simulink model "test02"  (R2025b)
settings: Solver=VariableStepAuto  StartTime=0.0  StopTime=60  RelTol=1e-3
settings Model: Creator=sanborkl  LastModifiedBy=sanborkl

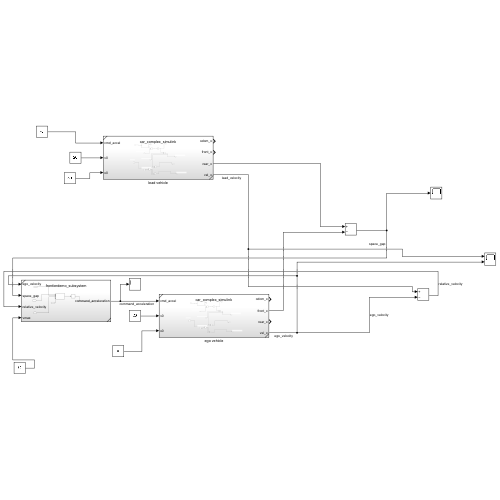
[thumbnail: Simulink's stored preview of the top-level diagram]
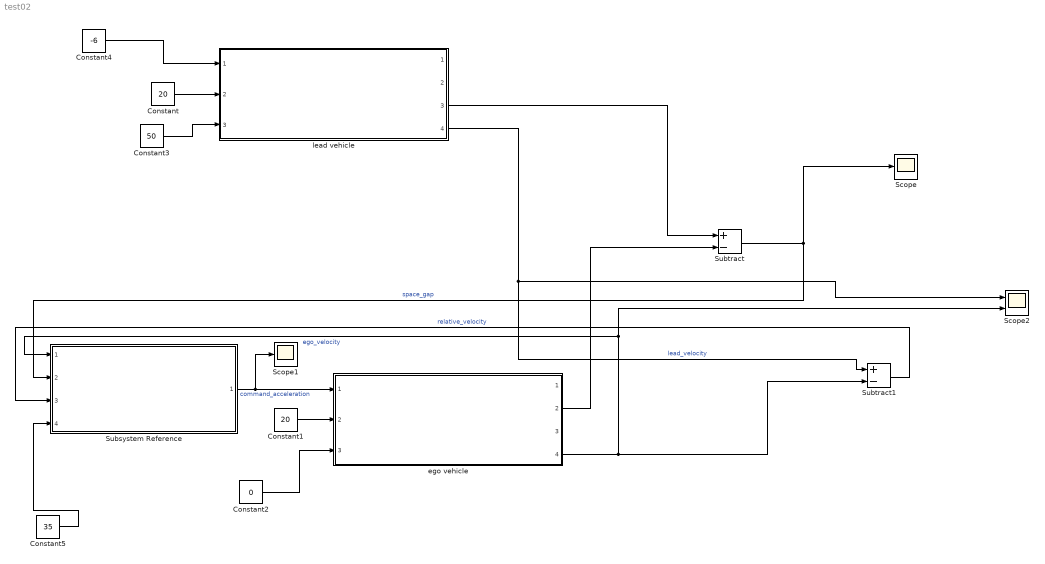
== system test02 ==
  Constant : Constant  Value=20
  Constant1 : Constant  Value=20
  Constant2 : Constant  Value=0
  Constant3 : Constant  Value=50
  Constant4 : Constant  Value=-6
  Constant5 : Constant  Value=35
  Scope : Scope
      settings: ActiveDisplayYMinimum=5.5000025780209976  ActiveDisplayYMaximum=50.499999713553223
  Scope1 : Scope
      settings: ActiveDisplayYMinimum=-2.7488890529903189  ActiveDisplayYMaximum=0.30543199948463784
  Scope2 : Scope  NumInputPorts=2
      settings: ActiveDisplayYMinimum=-2.4999999999999996  ActiveDisplayYMaximum=22.5  DataLoggingVariableName=ScopeData2
  Subsystem Reference : Subsystem  ReferencedSubsystem=frontierdemo_subsystem
  Subtract : Sum  Inputs=+-
  Subtract1 : Sum  Inputs=+-
  ego vehicle : Subsystem  ReferencedSubsystem=car_complex_simulink
  lead vehicle : Subsystem  ReferencedSubsystem=car_complex_simulink
  wires:
  Constant4/1 -> lead vehicle/1
  ego vehicle/2 -> Subtract/2
  Constant3/1 -> lead vehicle/3
  Subsystem Reference/1 -> Scope1/1, ego vehicle/1  "command_acceleration"
  Subtract/1 -> Subsystem Reference/2, Scope/1  "space_gap"
  Constant/1 -> lead vehicle/2
  Subtract1/1 -> Subsystem Reference/3  "relative_velocity"
  Constant1/1 -> ego vehicle/2
  lead vehicle/3 -> Subtract/1
  lead vehicle/4 -> Scope2/1, Subtract1/1  "lead_velocity"
  ego vehicle/4 -> Scope2/2, Subsystem Reference/1, Subtract1/2  "ego_velocity"
  Constant2/1 -> ego vehicle/3
  Constant5/1 -> Subsystem Reference/4
